simulink subsystem "LQR_tracking"  (R2024a)
settings: Solver=VariableStepAuto  StartTime=0.0  StopTime=10.0  RelTol=1e-3
undefined symbols (not defined in the file): K_LQR_tracking
settings Model: Creator=Bocchio  LastModifiedBy=Bocchio

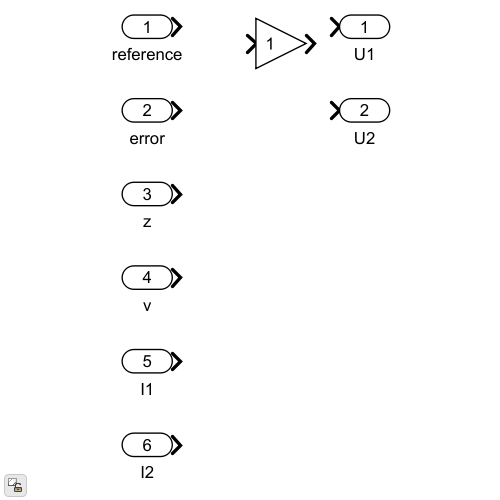
[thumbnail: Simulink's stored preview of the top-level diagram]
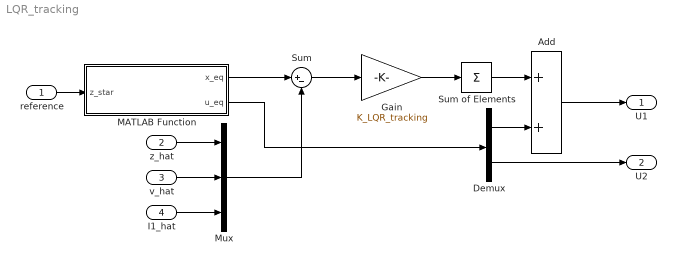
== system LQR_tracking ==
  reference : Inport
  z_hat : Inport  Port=2
  v_hat : Inport  Port=3
  I1_hat : Inport  Port=4
  Add : Sum
  Demux : Demux  Outputs=2
  Gain : Gain  Gain=K_LQR_tracking
  MATLAB Function : MATLAB Function  TreatAsAtomicUnit=on
  Mux : Mux  Inputs=3
  Sum : Sum  Inputs=|+-
  Sum of Elements : Sum  Inputs=+
  U1 : Outport
  U2 : Outport  Port=2
  wires:
  I1_hat/1 -> Mux/3
  v_hat/1 -> Mux/2
  z_hat/1 -> Mux/1
  Mux/1 -> Sum/2
  Sum/1 -> Gain/1
  Gain/1 -> Sum of Elements/1
  Sum of Elements/1 -> Add/1
  Add/1 -> U1/1
  MATLAB Function/2(u_eq) -> Demux/1
  Demux/1 -> Add/2
  Demux/2 -> U2/1
  reference/1 -> MATLAB Function/1(z_star)
  MATLAB Function/1(x_eq) -> Sum/1

== matlab function LQR_tracking/MATLAB Function ==
  data: z_star input; x_eq output; u_eq output
function [x_eq, u_eq] = operating_point(z_star)

g   = 9.81; %[m/s^2]
H = 98.00 * 1e-3; %[m]
m = 60.54 * 1e-3;   %[kg]
r = 61.25/2 * 1e-3; %[m]

I1min = 2.383122e-02; %[A]
I2min = 2.591441e-02; %[A]
k1 = +1.165800e+01; %[V/MU]
k2 = +1.165800e+01; %[V/MU]

a1z = 1.837302e+02; %[1/m]
a2z = 1.837302e+02; %[1/m]
L1z = 3.438228e-02; %[H]
L2z = 3.438228e-02; %[H]

R10 = 4.17; %[ohm]
R20 = 4.20; %[ohm]

dL1dx = @(x) -a1z*L1z * exp(-a1z*x);
dL2dx = @(x) +a2z*L2z * exp(-a2z*(H - 2*r - x));

x_eq = zeros(3, 1)';
u_eq = zeros(2, 1);

x_eq(1) = z_star;
x_eq(2) = 0;
x_eq(3) = sqrt( -(2*m*g + dL2dx(x_eq(1)) * I2min^2) / dL1dx(x_eq(1)) );

u_eq(1) = max([0, R10 * (x_eq(3) - I1min) / k1]);
u_eq(2) = 0;

end
